simulink subsystem "SMC_Test"  (R2026a)
settings: Solver=VariableStepAuto
libraries: simulink x1
settings Model: Creator=maxim  LastModifiedBy=maxim

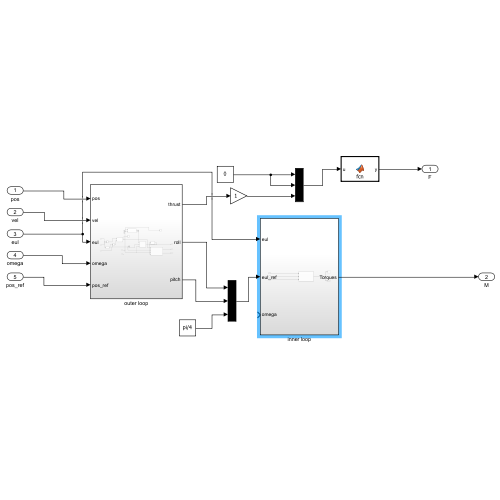
[thumbnail: Simulink's stored preview of the top-level diagram]
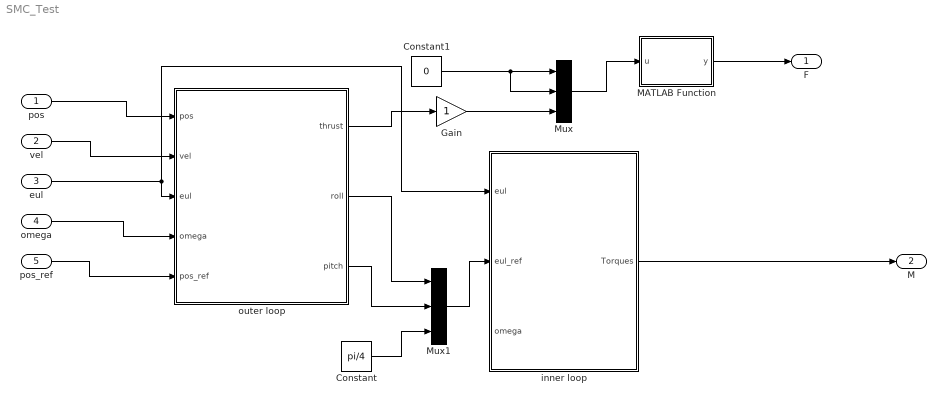
== system SMC_Test ==
  pos : Inport
  vel : Inport  Port=2
  eul : Inport  Port=3
  omega : Inport  Port=4
  pos_ref : Inport  Port=5
  Constant : Constant  Value=pi/4
  Constant1 : Constant  Value=0
  Gain : Gain
  MATLAB Function : MATLAB Function  TreatAsAtomicUnit=on
  Mux : Mux  Inputs=3
  Mux1 : Mux  Inputs=3
  inner loop : Subsystem
  outer loop : Subsystem
  F : Outport
  M : Outport  Port=2
  wires:
  Constant/1 -> Mux1/3
  outer loop/2(roll) -> Mux1/1
  outer loop/1(thrust) -> Gain/1
  pos/1 -> outer loop/1(pos)
  Gain/1 -> Mux/3
  Mux1/1 -> inner loop/2(eul_ref)
  MATLAB Function/1(y) -> F/1
  eul/1 -> outer loop/3(eul), inner loop/1(eul)
  Constant1/1 -> Mux/1, Mux/2
  pos_ref/1 -> outer loop/5(pos_ref)
  inner loop/1(Torques) -> M/1
  vel/1 -> outer loop/2(vel)
  outer loop/3(pitch) -> Mux1/2
  omega/1 -> outer loop/4(omega)
  Mux/1 -> MATLAB Function/1(u)

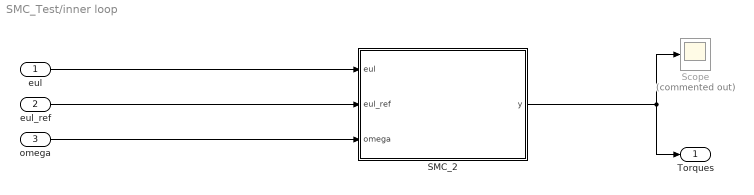
== system SMC_Test/inner loop ==
  eul : Inport
  eul_ref : Inport  Port=2
  omega : Inport  Port=3
  SMC_2 : MATLAB Function  TreatAsAtomicUnit=on
  Scope : Scope  Commented=on
      settings: ActiveDisplayYMinimum=-0.0018422520455562647  ActiveDisplayYMaximum=0.0038643170015684822  DataLoggingVariableName=ScopeData2
  Torques : Outport
  wires:
  SMC_2/1(y) -> Torques/1, Scope/1
  eul/1 -> SMC_2/1(eul)
  eul_ref/1 -> SMC_2/2(eul_ref)
  omega/1 -> SMC_2/3(omega)

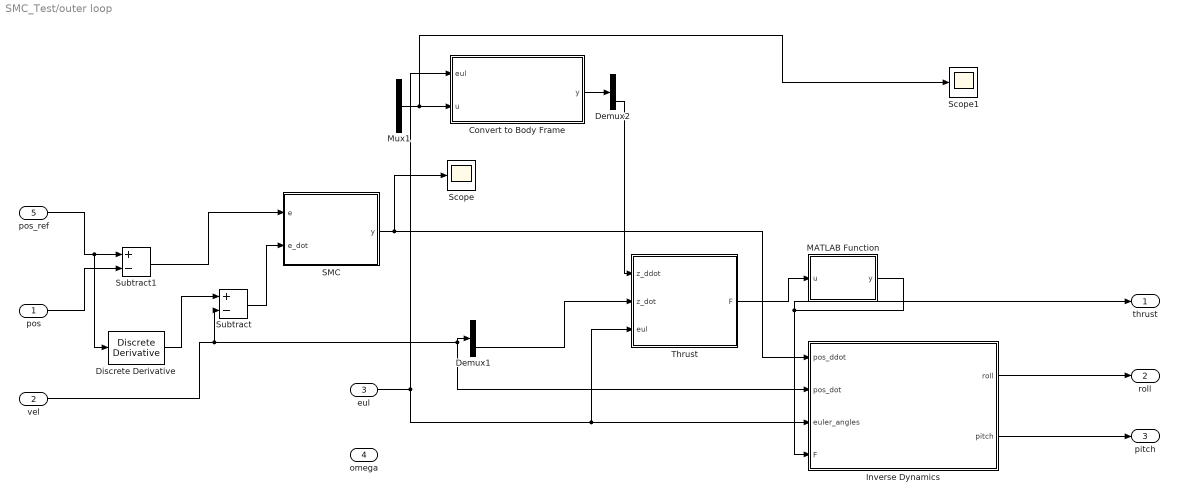
== system SMC_Test/outer loop ==
  pos : Inport
  vel : Inport  Port=2
  eul : Inport  Port=3
  omega : Inport  Port=4
  pos_ref : Inport  Port=5
  Convert to Body Frame : MATLAB Function  TreatAsAtomicUnit=on
  Demux1 : Demux  Outputs=3
  Demux2 : Demux  Outputs=3
  Discrete Derivative : simulink/Discrete/Discrete Derivative  gainval=1.0  ICPrevScaledInput=0.0  OutMin=[]  OutMax=[]  OutDataType=fixdt(1, 16)  OutScaling=2^-10  DoSatur=off
  Inverse Dynamics : MATLAB Function  TreatAsAtomicUnit=on
  MATLAB Function : MATLAB Function  TreatAsAtomicUnit=on
  Mux1 : Mux  Inputs=3
  SMC : MATLAB Function  TreatAsAtomicUnit=on
  Scope : Scope
  Scope1 : Scope
      settings: ActiveDisplayYMinimum=-0.14545123162876328  ActiveDisplayYMaximum=0.14023265670551954  DataLoggingVariableName=ScopeData3
  Subtract : Sum  Inputs=+-
  Subtract1 : Sum  Inputs=+-
  Thrust : MATLAB Function  TreatAsAtomicUnit=on
  thrust : Outport
  roll : Outport  Port=2
  pitch : Outport  Port=3
  wires:
  eul/1 -> Convert to Body Frame/1(eul), Thrust/3(eul), Inverse Dynamics/3(euler_angles)
  Demux1/3 -> Thrust/2(z_dot)
  MATLAB Function/1(y) -> thrust/1, Inverse Dynamics/4(F)
  Inverse Dynamics/1(roll) -> roll/1
  Inverse Dynamics/2(pitch) -> pitch/1
  pos_ref/1 -> Discrete Derivative/1, Subtract1/1
  Mux1/1 -> Scope1/1, Convert to Body Frame/2(u)
  Convert to Body Frame/1(y) -> Demux2/1
  Demux2/3 -> Thrust/1(z_ddot)
  Thrust/1(F) -> MATLAB Function/1(u)
  pos/1 -> Subtract1/2
  vel/1 -> Subtract/2, Demux1/1, Inverse Dynamics/2(pos_dot)
  SMC/1(y) -> Inverse Dynamics/1(pos_ddot), Scope/1
  Discrete Derivative/1 -> Subtract/1
  Subtract/1 -> SMC/2(e_dot)
  Subtract1/1 -> SMC/1(e)

== matlab function SMC_Test/outer loop/SMC ==
  data: e input; y output; e_dot input
function y = SMC(e, e_dot)

% Tuning parameters
lambda = [1.5; 1.5; 1.2];
K      = [2.0; 2.0; 1.5];
phi    = [0.25; 0.25; 0.25];
a_max  = [3.0; 3.0; 2.0];

% Sliding surface
s = e_dot + lambda .* e;

% Smooth saturation function, limited to [-1, 1]
sat_s = max(-ones(3,1), min(ones(3,1), s ./ phi));

% SMC desired-acceleration command
y = lambda .* e_dot + K .* sat_s;

% Acceleration safety limits
y = max(-a_max, min(a_max, y));
end

== matlab function SMC_Test/outer loop/Inverse Dynamics ==
  data: roll output; pitch output; pos_ddot input; pos_dot input; euler_angles input; F input
function [roll, pitch] = inverse_dynamics(pos_ddot, pos_dot, euler_angles, F)
    [r, p] = solve_roll_pitch(pos_ddot, pos_dot, euler_angles, F);
    roll = clip(r, -0.5, 0.5);
    pitch = clip(p, -0.5, 0.5);

== matlab function SMC_Test/inner loop/SMC_2 ==
  data: eul input; eul_ref input; y output; omega input
function y = SMC_2(eul, eul_ref, omega)
% y = [Mx; My; Mz] torque commands, N*m

lambda = [6; 6; 3];
K      = [0.08; 0.08; 0.03];
phi    = [0.08; 0.08; 0.05];
M_max  = [0.10; 0.10; 0.04];

% Wrapped measured-minus-reference attitude error
e = atan2(sin(eul - eul_ref), cos(eul - eul_ref));

% Sliding surface: angular-rate damping + angle correction
s = omega + lambda .* e;

% Smooth SMC switching function
sat_s = max(-ones(3,1), min(ones(3,1), s ./ phi));

% Corrective moment command
y = -K .* sat_s;

% Moment safety limits
y = max(-M_max, min(M_max, y));
end

== matlab function SMC_Test/outer loop/Thrust ==
  data: z_ddot input; F output; z_dot input; eul input
function F = thrust(z_ddot, z_dot, eul)
    F = solve_thrust(z_ddot, z_dot, eul);

== matlab function SMC_Test/outer loop/Convert to Body Frame ==
  data: eul input; u input; y output
function y = convert_to_body(eul, u)
    R = eul2rotm([eul(3), eul(2), eul(1)]);
    y = R' * u;

== matlab function SMC_Test/MATLAB Function ==
  data: u input; y output
function y = fcn(u)
    
y = clip(u, 0, 20);

== matlab function SMC_Test/outer loop/MATLAB Function ==
  data: u input; y output
function y = fcn(u)
    
y = clip(u, 1, 20);
